simulink model "pid_test2"  (R2019b)
settings: Solver=FixedStepAuto  StartTime=0.0  StopTime=10  FixedStep=0.001  RelTol=1e-3
settings Model: Creator=subhgang  LastModifiedBy=subhgang

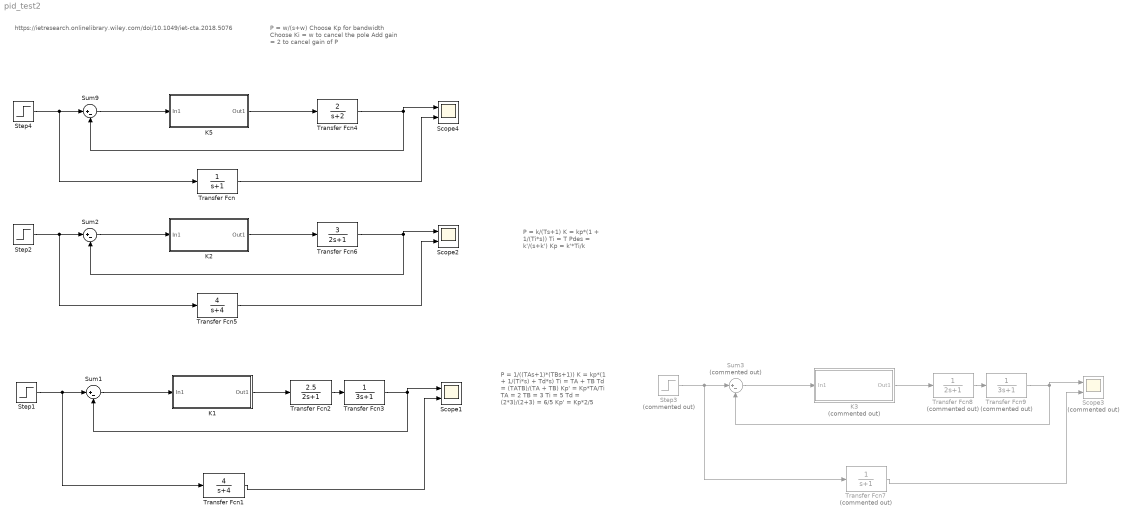
== system pid_test2 ==
  note: https://ietresearch.onlinelibrary.wiley.com/doi/10.1049/iet-cta.2018.5076
  note: P = 1/((TAs+1)*(TBs+1))
      |
      | K = kp*(1 + 1/(Ti*s) + Td*s)
      |
      | Ti = TA + TB
      | Td = (TATB)/(TA + TB)
      | Kp' = Kp*TA/Ti
      |
      | TA = 2
      | TB = 3
      |
      | Ti = 5
      | Td = (2*3)/(2+3) = 6/5
      | Kp' = Kp*2/5
  note: P = w/(s+w)
      |
      | Choose Kp for bandwidth
      | Choose Ki = w to cancel the pole
      |
      | Add gain = 2 to cancel gain of P
  note: P = k/(Ts+1)
      |
      | K = kp*(1 + 1/(Ti*s))
      |
      | Ti = T
      |
      | Pdes = k'/(s+k')
      |
      | Kp = k'*Ti/k
  K1 : Subsystem
  K2 : Subsystem
  K3 : Subsystem  Commented=on
  K5 : Subsystem
  Scope1 : Scope  NumInputPorts=2
  Scope2 : Scope  NumInputPorts=2
  Scope3 : Scope  Commented=on  NumInputPorts=2
  Scope4 : Scope  NumInputPorts=2
  Step1 : Step  SampleTime=0
  Step2 : Step  SampleTime=0
  Step3 : Step  Commented=on  SampleTime=0
  Step4 : Step  SampleTime=0
  Sum1 : Sum  Inputs=|+-
  Sum2 : Sum  Inputs=|+-
  Sum3 : Sum  Commented=on  Inputs=|+-
  Sum9 : Sum  Inputs=|+-
  Transfer Fcn : TransferFcn  Denominator=[1 1]
  Transfer Fcn1 : TransferFcn  Numerator=[4]  Denominator=[1 4]
  Transfer Fcn2 : TransferFcn  Numerator=[2.5]  Denominator=[2 1]
  Transfer Fcn3 : TransferFcn  Denominator=[3 1]
  Transfer Fcn4 : TransferFcn  Numerator=[2]  Denominator=[1 2]
  Transfer Fcn5 : TransferFcn  Numerator=[4]  Denominator=[1 4]
  Transfer Fcn6 : TransferFcn  Numerator=[3]  Denominator=[2 1]
  Transfer Fcn7 : TransferFcn  Commented=on  Denominator=[1 1]
  Transfer Fcn8 : TransferFcn  Commented=on  Denominator=[2 1]
  Transfer Fcn9 : TransferFcn  Commented=on  Denominator=[3 1]
  wires:
  K5/1(Out1) -> Transfer Fcn4/1
  Sum9/1 -> K5/1(In1)
  Step4/1 -> Transfer Fcn/1, Sum9/1
  Transfer Fcn4/1 -> Scope4/1, Sum9/2
  Transfer Fcn/1 -> Scope4/2
  K1/1(Out1) -> Transfer Fcn2/1
  Step1/1 -> Transfer Fcn1/1, Sum1/1
  Transfer Fcn2/1 -> Transfer Fcn3/1
  Sum1/1 -> K1/1(In1)
  Transfer Fcn1/1 -> Scope1/2
  Transfer Fcn3/1 -> Scope1/1, Sum1/2
  K2/1(Out1) -> Transfer Fcn6/1
  Step2/1 -> Transfer Fcn5/1, Sum2/1
  Transfer Fcn6/1 -> Scope2/1, Sum2/2
  Sum2/1 -> K2/1(In1)
  Transfer Fcn5/1 -> Scope2/2
  Transfer Fcn8/1 -> Transfer Fcn9/1
  Sum3/1 -> K3/1(In1)
  Transfer Fcn7/1 -> Scope3/2
  Step3/1 -> Transfer Fcn7/1, Sum3/1
  K3/1(Out1) -> Transfer Fcn8/1
  Transfer Fcn9/1 -> Scope3/1, Sum3/2

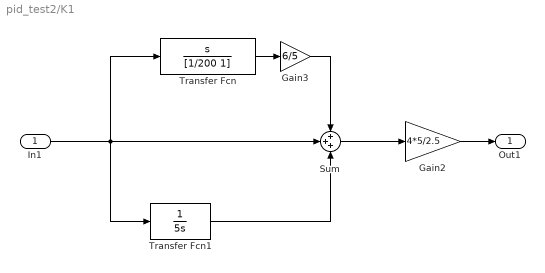
== system pid_test2/K1 ==
  In1 : Inport
  Gain2 : Gain  Gain=4*5/2.5
  Gain3 : Gain  Gain=6/5
  Sum : Sum  Inputs=+++
  Transfer Fcn : TransferFcn  Numerator=[1 0]  Denominator=[1/200 1]
  Transfer Fcn1 : TransferFcn  Denominator=[5 0]
  Out1 : Outport
  wires:
  Sum/1 -> Gain2/1
  Gain2/1 -> Out1/1
  Transfer Fcn/1 -> Gain3/1
  In1/1 -> Transfer Fcn1/1, Sum/2, Transfer Fcn/1
  Transfer Fcn1/1 -> Sum/3
  Gain3/1 -> Sum/1

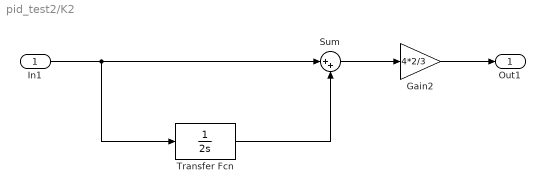
== system pid_test2/K2 ==
  In1 : Inport
  Gain2 : Gain  Gain=4*2/3
  Sum : Sum  Inputs=|++
  Transfer Fcn : TransferFcn  Denominator=[2 0]
  Out1 : Outport
  wires:
  In1/1 -> Transfer Fcn/1, Sum/1
  Sum/1 -> Gain2/1
  Gain2/1 -> Out1/1
  Transfer Fcn/1 -> Sum/2

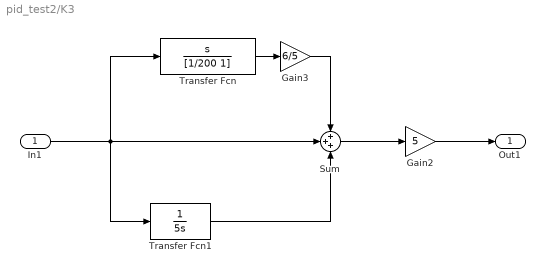
== system pid_test2/K3 ==
  In1 : Inport
  Gain2 : Gain  Gain=5
  Gain3 : Gain  Gain=6/5
  Sum : Sum  Inputs=+++
  Transfer Fcn : TransferFcn  Numerator=[1 0]  Denominator=[1/200 1]
  Transfer Fcn1 : TransferFcn  Denominator=[5 0]
  Out1 : Outport
  wires:
  Sum/1 -> Gain2/1
  Gain2/1 -> Out1/1
  Transfer Fcn/1 -> Gain3/1
  In1/1 -> Transfer Fcn1/1, Sum/2, Transfer Fcn/1
  Transfer Fcn1/1 -> Sum/3
  Gain3/1 -> Sum/1

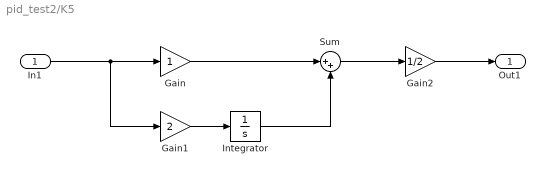
== system pid_test2/K5 ==
  In1 : Inport
  Gain : Gain
  Gain1 : Gain  Gain=2
  Gain2 : Gain  Gain=1/2
  Integrator : Integrator
  Sum : Sum  Inputs=|++
  Out1 : Outport
  wires:
  In1/1 -> Gain1/1, Gain/1
  Gain1/1 -> Integrator/1
  Gain/1 -> Sum/1
  Integrator/1 -> Sum/2
  Sum/1 -> Gain2/1
  Gain2/1 -> Out1/1
